simulink model "DesignProject"  (R2024b)
settings: Solver=VariableStepAuto  StartTime=0.0  StopTime=10.0  RelTol=1e-3
libraries: simulink_extras x7, simulink x1
settings Model: Creator=ryans  LastModifiedBy=ryans

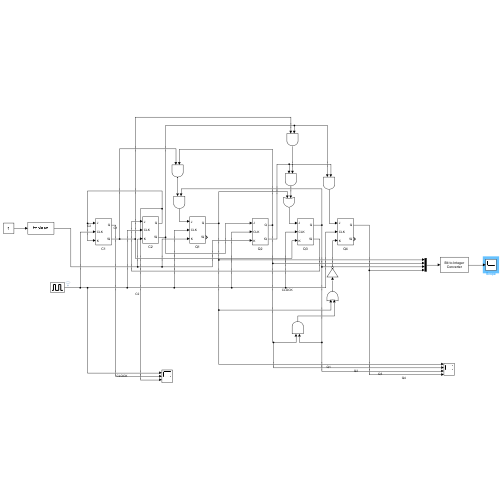
[thumbnail: Simulink's stored preview of the top-level diagram]
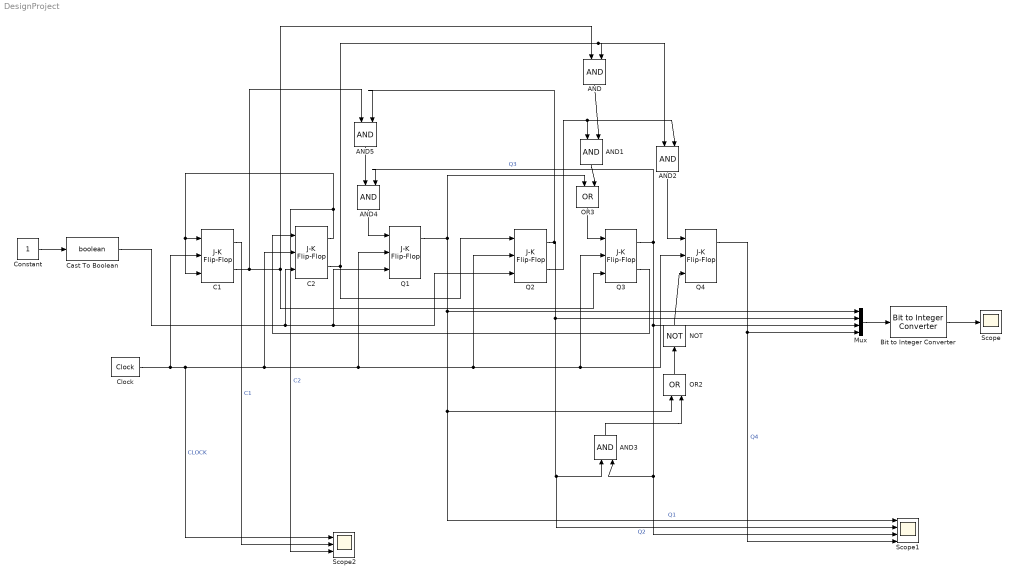
== system DesignProject ==
  AND{,1..5} (6 alike) : Logic  IconShape=distinctive  AllPortsSameDT=off  OutDataTypeStr=boolean
  Bit to Integer Converter : simulink/Logic and Bit Operations/Bit to Integer Converter  nbits=4  bitOrder=MSB first  signedOutputValues=Unsigned  outDtype=Inherit via internal rule  outDtypeSigned=Inherit via internal rule
  C1 : simulink_extras/Flip Flops/J-K Flip-Flop  initial_condition=0
  C2 : simulink_extras/Flip Flops/J-K Flip-Flop  initial_condition=0
  Cast To Boolean : DataTypeConversion  OutDataTypeStr=boolean  SaturateOnIntegerOverflow=off  RndMeth=Floor
  Clock : simulink_extras/Flip Flops/Clock  period=0.4
  Constant : Constant
  Mux : Mux
  NOT : Logic  Operator=NOT  IconShape=distinctive  AllPortsSameDT=off  OutDataTypeStr=boolean
  OR2 : Logic  Operator=OR  IconShape=distinctive  AllPortsSameDT=off  OutDataTypeStr=boolean
  OR3 : Logic  Operator=OR  IconShape=distinctive  AllPortsSameDT=off  OutDataTypeStr=boolean
  Q1 : simulink_extras/Flip Flops/J-K Flip-Flop  initial_condition=0
  Q2 : simulink_extras/Flip Flops/J-K Flip-Flop  initial_condition=1
  Q3 : simulink_extras/Flip Flops/J-K Flip-Flop  initial_condition=0
  Q4 : simulink_extras/Flip Flops/J-K Flip-Flop  initial_condition=0
  Scope : Scope
  Scope1 : Scope  NumInputPorts=4
  Scope2 : Scope  NumInputPorts=3
  wires:
  Clock/1 -> Scope2/1, Q4/2, Q3/2, Q2/2, Q1/2, C2/2, C1/2  "CLOCK"
  Q4/1 -> Scope1/4, Mux/4  "Q4"
  C1/2 -> AND5/1, Q3/3, AND/1
  Q3/1 -> AND4/2, Scope1/3, AND3/2, Mux/3  "Q3"
  AND5/1 -> AND4/1
  C2/2 -> AND2/1, AND/2, Q2/1
  Q2/2 -> AND2/2, AND1/1
  AND/1 -> AND1/2
  AND2/1 -> Q4/1
  Q2/1 -> AND5/2, Mux/2, Scope1/2, AND3/1  "Q2"
  Q3/2 -> C2/1
  Q1/1 -> OR3/1, Mux/1, OR2/1, Scope1/1  "Q1"
  AND3/1 -> OR2/2
  OR2/1 -> NOT/1
  NOT/1 -> Q4/3
  C2/1 -> Scope2/3, C1/1, C1/3  "C2"
  Constant/1 -> Cast To Boolean/1
  Cast To Boolean/1 -> Q1/3, Q2/3, C2/3
  Mux/1 -> Bit to Integer Converter/1
  Bit to Integer Converter/1 -> Scope/1
  AND4/1 -> Q1/1
  AND1/1 -> OR3/2
  OR3/1 -> Q3/1
  C1/1 -> Scope2/2  "C1"
